simulink model "EIRSAT_ADCS"  (R2017a)
settings: Solver=ode45  StartTime=0.0  StopTime=T_stop  RelTol=1e-6
values from neighbouring files (symbols this model uses):
  aerodrag_A_d = 0.2*0.1*sqrt(2)    [Satellite_Setup.m]
  aerodrag_c_p = 0.02*[1;1;1]    [Satellite_Setup.m]
  I = diag([Ixx;Iyy;Izz])    [Satellite_Setup.m]
  igrf_L = 10    [Satellite_Setup.m]
  igrf_tol = 1e-9    (= 1e-09)    [Satellite_Setup.m]
  mass = 2.6    [Satellite_Setup.m]
  omega_orbit = [0;-7.67/(401.1+6371);0]    [Satellite_Setup.m]
undefined symbols (not defined in the file or in its folder): control_tolerance, distrej, igrf_G, igrf_H, k, kd, kp, nAx, nAy, nAz, q_ref, x_0, x_orbit_init
libraries: cstblocks x12, sharedtransform x4
settings Model: Creator=JoeT  LastModifiedBy=vicctorio
settings DataIOCC: LimitDataPoints=on  SaveFormat=Array
settings OptimizationCC: BlockReduction=off  BooleanDataType=off  LifeSpan=inf
settings DebuggingCC: SaveWithParameterizedLinksMsg=none  UnderspecifiedInitializationDetection=Classic  MergeDetectMultiDrivingBlocksExec=none  SignalResolutionControl=TryResolveAllWithWarning  SFUnexpectedBacktrackingDiag=warning  SFNoUnconditionalDefaultTransitionDiag=warning  SFExecutionAtInitializationDiag=none
settings HardwareCC: ProdBitPerPointer=32  ProdBitPerSizeT=32  ProdBitPerPtrDiffT=32  ProdLargestAtomicFloat=None  ProdIntDivRoundTo=Undefined  ProdEndianess=Unspecified  ProdWordSize=32  ProdHWDeviceType=32-bit Generic  TargetUnknown=on
settings ModelReferenceCC: PropagateSignalLabelsOutOfModel=off
settings GRTTargetCC: TargetLangStandard=C89/C90 (ANSI)  GeneratePreprocessorConditionals=Disable all
settings ConfigComp: CovMetricSettings=dw  CovHtmlReporting=on  CovSaveCumulativeToWorkspaceVar=on  CovSaveSingleToWorkspaceVar=on  CovExternalEMLEnable=off  CovSFcnEnable=off

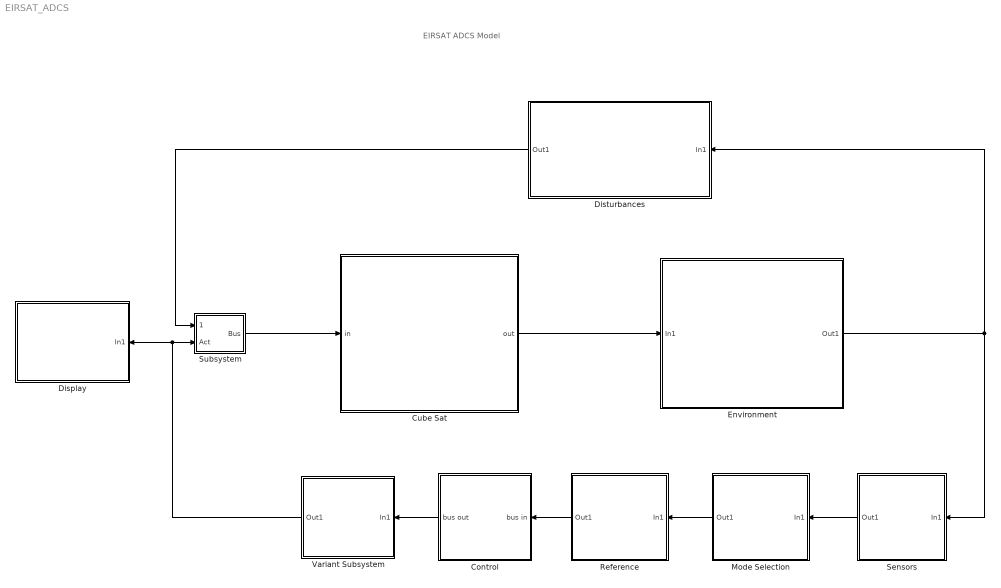
== system EIRSAT_ADCS ==
  note: EIRSAT ADCS Model
  Control : Subsystem  Variant=on
  Cube Sat : Subsystem
  Display : Subsystem
  Disturbances : Subsystem
  Environment : Subsystem
  Mode Selection : Subsystem
  Reference : Subsystem
  Sensors : Subsystem
  Subsystem : Subsystem
  Variant Subsystem : Subsystem  Variant=on
  wires:
  Mode Selection/1(Out1) -> Reference/1(In1)
  Sensors/1(Out1) -> Mode Selection/1(In1)
  Reference/1(Out1) -> Control/1(bus in)
  Control/1(bus out) -> Variant Subsystem/1(In1)
  Disturbances/1(Out1) -> Subsystem/1(Disturb)
  Cube Sat/1(out) -> Environment/1(In1)
  Environment/1(Out1) -> Sensors/1(In1), Disturbances/1(In1)
  Variant Subsystem/1(Out1) -> Subsystem/2(Act), Display/1(In1)
  Subsystem/1(Bus) -> Cube Sat/1(in)

== system EIRSAT_ADCS/Control ==
  note: 1) Only subsystems can be added as variant choices at this level
      | 2) Blocks cannot be connected at this level as connectivity is
      | automatically determined at simulation, based on the active variant
  bus in : Inport
  PD : Subsystem  VariantControl=CtrlType==2
  WBC : Subsystem  VariantControl=CtrlType==1
  no control : Subsystem  VariantControl=CtrlType==0
  bus out : Outport

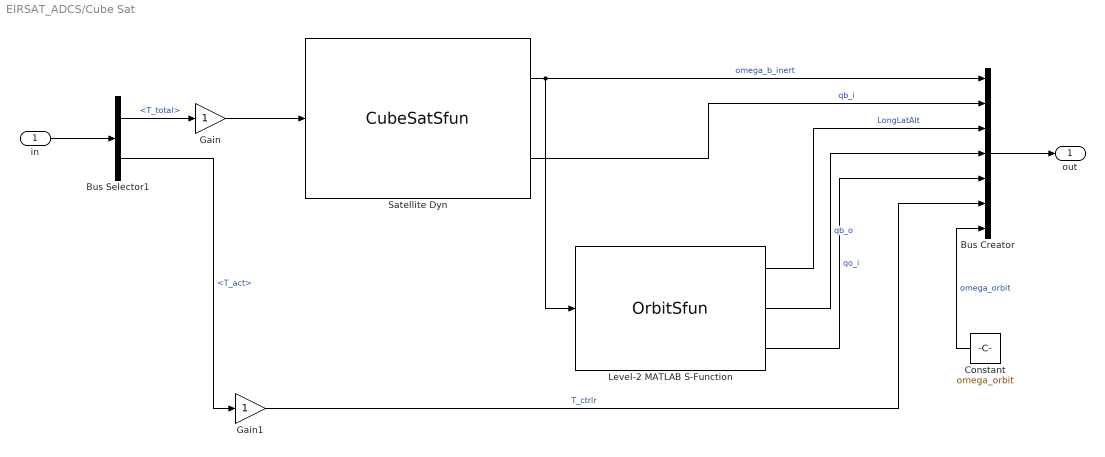
== system EIRSAT_ADCS/Cube Sat ==
  in : Inport
  Bus Creator : BusCreator  Inputs=7
  Bus Selector1 : BusSelector  OutputSignals=T_total,T_act
  Constant : Constant  Value=omega_orbit
  Gain : Gain
  Gain1 : Gain
  Level-2 MATLAB S-Function : M-S-Function  FunctionName=OrbitSfun  Parameters=x_orbit_init,omega_orbit  mask{Parameter1=x_orbit_init, Parameter2=omega_orbit}
      mask prompts: Parameter1 "Initial orbit param"; Parameter2 "orbit angular velocity"
      mask DialogControl Control8 Prompt: Orbit properties
      mask Display:
      | disp('Orbital Parameters')
      | port_label('input',1,'ang vel')
      | port_label('output',1,'LLA')
      | port_label('output',2,'qb_o')
      | port_label('output',3,'qo_i')
  Satellite Dyn : M-S-Function  FunctionName=CubeSatSfun  Parameters=x_0,I  mask{Parameter2=x_0, Parameter3=I}
      mask prompts: Parameter2 "x_0"; Parameter3 "I"
      mask DialogControl DescTextVar Prompt: Model of a rigid CubeSat. Model takes Torque about each axis as an input. The first output is the angular velocity of the sat wrt an inertial frame. The second output is the quaternion which represents the rotation between inertial and body fixed frames
      mask Display:
      | disp('Cube Sat Model')
      | port_label('input',1,'Torq')
      | port_label('output',1,'Ang Vel')
      | port_label('output',2,'Quat')
  out : Outport
  wires:
  Bus Creator/1 -> out/1
  in/1 -> Bus Selector1/1
  Bus Selector1/1 -> Gain/1  "<T_total>"
  Satellite Dyn/1 -> Level-2 MATLAB S-Function/1, Bus Creator/1  "omega_b_inert"
  Gain/1 -> Satellite Dyn/1
  Satellite Dyn/2 -> Bus Creator/2  "qb_i"
  Level-2 MATLAB S-Function/1 -> Bus Creator/3  "LongLatAlt"
  Level-2 MATLAB S-Function/2 -> Bus Creator/4  "qb_o"
  Level-2 MATLAB S-Function/3 -> Bus Creator/5  "qo_i"
  Constant/1 -> Bus Creator/7  "omega_orbit"
  Bus Selector1/2 -> Gain1/1  "<T_act>"
  Gain1/1 -> Bus Creator/6  "T_ctrlr"

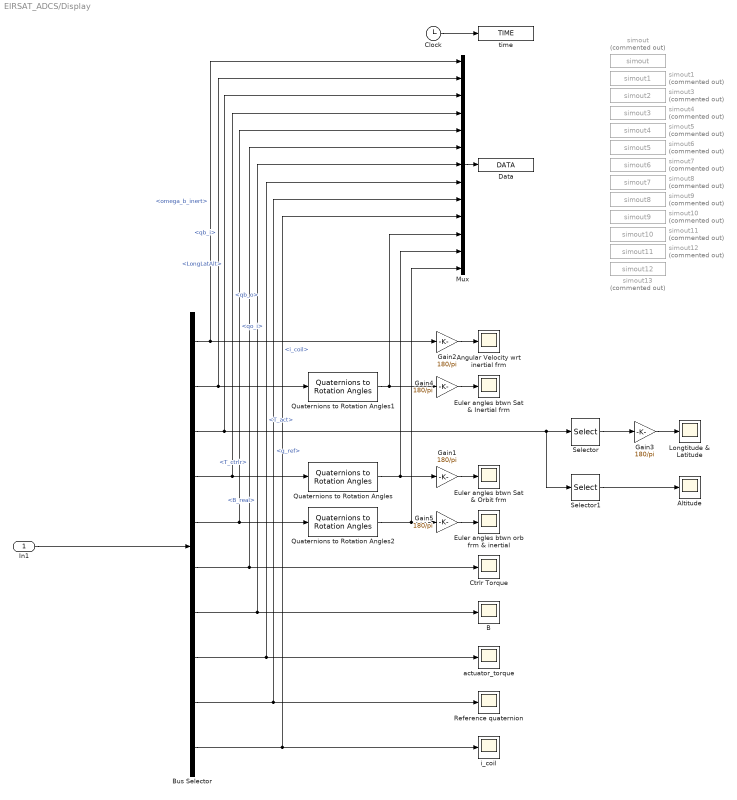
== system EIRSAT_ADCS/Display ==
  In1 : Inport
  Altitude : Scope
  Angular Velocity wrt inertial frm : Scope
  B : Scope
  Bus Selector : BusSelector  OutputSignals=Ctrlr_out.ref_out.signal1.Sensor_out.Enviro_out.Dyn_out.omega_b_inert,Ctrlr_out.ref_out.signal1.Sensor_out.Enviro_out.Dyn_out.qb_i,Ctrlr_out.ref_out.signal1.Sensor_out.Enviro_out.Dyn_out.LongLatAlt,Ctrlr_out.ref_out.signal1.Sensor_out.Enviro_out.Dyn_out.qb_o,Ctrlr_out.ref_out.signal1.Sensor_out.Enviro_out.Dyn_out.qo_i,Ctrlr_out.ref_out.signal1.Sensor_out.Enviro_out.Dyn_out.T_ctrlr,Ctrlr_out.ref_out.signal1.Sensor_out.Sensor_values.B_real,T_act,Ctrlr_out.ref_out.q_ref,i_coil
  Clock : Clock
  Ctrlr Torque : Scope
  "Data " : ToWorkspace  VariableName=DATA  SampleTime=-1
  Euler angles btwn Sat & Inertial frm : Scope
  Euler angles btwn Sat & Orbit frm : Scope
  Euler angles btwn orb frm & inertial : Scope
  Gain{1..5} (5 alike) : Gain  Gain=180/pi
  Longtitude & Latitude : Scope
  Mux : Mux  Inputs=13
  Quaternions to Rotation Angles : sharedtransform/Quaternions to Rotation Angles  rotationOrder=XYZ
  Quaternions to Rotation Angles1 : sharedtransform/Quaternions to Rotation Angles  rotationOrder=XYZ
  Quaternions to Rotation Angles2 : sharedtransform/Quaternions to Rotation Angles  rotationOrder=XYZ
  Reference quaternion : Scope
  Selector : Selector  InputPortWidth=3  IndexOptions=Index vector (dialog)  Indices=[1 2]  OutputSizes=1
  Selector1 : Selector  InputPortWidth=3  IndexOptions=Index vector (dialog)  Indices=[3]  OutputSizes=1
  actuator_torque : Scope
  i_coil : Scope
  "simout " : ToWorkspace  Commented=on  VariableName=simout  SaveFormat=Timeseries  SampleTime=-1
  simout1 : ToWorkspace  Commented=on  VariableName=simout1  SaveFormat=Timeseries  SampleTime=-1
  simout10 : ToWorkspace  Commented=on  VariableName=simout9  SaveFormat=Timeseries  SampleTime=-1
  simout11 : ToWorkspace  Commented=on  VariableName=simout10  SaveFormat=Timeseries  SampleTime=-1
  simout12 : ToWorkspace  Commented=on  VariableName=simout11  SaveFormat=Timeseries  SampleTime=-1
  simout13 : ToWorkspace  Commented=on  VariableName=simout12  SaveFormat=Timeseries  SampleTime=-1
  simout3 : ToWorkspace  Commented=on  VariableName=simout2  SaveFormat=Timeseries  SampleTime=-1
  simout4 : ToWorkspace  Commented=on  VariableName=simout3  SaveFormat=Timeseries  SampleTime=-1
  simout5 : ToWorkspace  Commented=on  VariableName=simout4  SaveFormat=Timeseries  SampleTime=-1
  simout6 : ToWorkspace  Commented=on  VariableName=simout5  SaveFormat=Timeseries  SampleTime=-1
  simout7 : ToWorkspace  Commented=on  VariableName=simout6  SaveFormat=Timeseries  SampleTime=-1
  simout8 : ToWorkspace  Commented=on  VariableName=simout7  SaveFormat=Timeseries  SampleTime=-1
  simout9 : ToWorkspace  Commented=on  VariableName=simout8  SaveFormat=Timeseries  SampleTime=-1
  time : ToWorkspace  VariableName=TIME  SampleTime=-1
  wires:
  In1/1 -> Bus Selector/1
  Bus Selector/6 -> Mux/6, Ctrlr Torque/1  "<T_ctrlr>"
  Bus Selector/4 -> Mux/4, Quaternions to Rotation Angles/1  "<qb_o>"
  Bus Selector/1 -> Mux/1, Gain2/1  "<omega_b_inert>"
  Quaternions to Rotation Angles/1 -> Mux/12, Gain1/1
  Gain2/1 -> Angular Velocity wrt inertial frm/1
  Gain1/1 -> Euler angles btwn Sat & Orbit frm/1
  Selector/1 -> Gain3/1
  Gain3/1 -> Longtitude & Latitude/1
  Bus Selector/2 -> Mux/2, Quaternions to Rotation Angles1/1  "<qb_i>"
  Selector1/1 -> Altitude/1
  Quaternions to Rotation Angles2/1 -> Mux/13, Gain5/1
  Gain5/1 -> Euler angles btwn orb frm & inertial/1
  Bus Selector/3 -> Mux/3, Selector1/1, Selector/1  "<LongLatAlt>"
  Bus Selector/7 -> Mux/7, B/1  "<B_real>"
  Bus Selector/8 -> Mux/8, actuator_torque/1  "<T_act>"
  Bus Selector/9 -> Mux/9, Reference quaternion/1  "<q_ref>"
  Bus Selector/10 -> Mux/10, i_coil/1  "<i_coil>"
  Gain4/1 -> Euler angles btwn Sat & Inertial frm/1
  Bus Selector/5 -> Mux/5, Quaternions to Rotation Angles2/1  "<qo_i>"
  Quaternions to Rotation Angles1/1 -> Mux/11, Gain4/1
  Mux/1 -> "Data "/1
  Clock/1 -> time/1

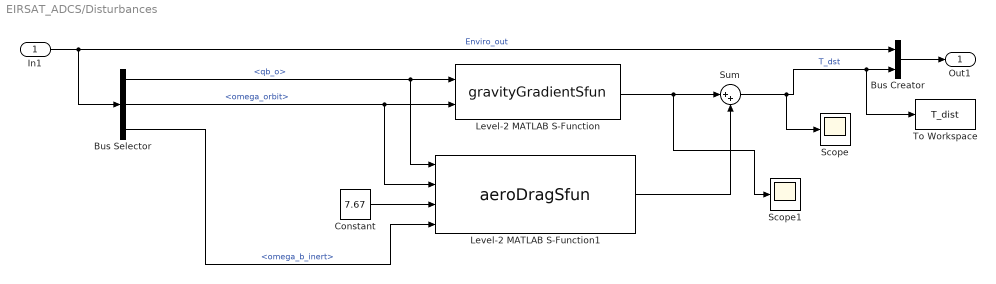
== system EIRSAT_ADCS/Disturbances ==
  In1 : Inport
  Bus Creator : BusCreator  Inputs=2
  Bus Selector : BusSelector  OutputSignals=Dyn_out.qb_o,Dyn_out.omega_orbit,Dyn_out.omega_b_inert
  Constant : Constant  Value=7.67
  Level-2 MATLAB S-Function : M-S-Function  FunctionName=gravityGradientSfun
      mask Display:
      | disp('Gravity\n gradient')
      | port_label('input',1,'qb_o')
      | port_label('input',2,'omega orbit')
      | port_label('output',1,'T_b')
  Level-2 MATLAB S-Function1 : M-S-Function  FunctionName=aeroDragSfun  Parameters=I,mass,aerodrag_c_p,aerodrag_A_d  mask{Parameter1=I, Parameter2=mass, Parameter3=aerodrag_c_p, Parameter4=aerodrag_A_d}
      mask prompts: Parameter1 "Inertia"; Parameter2 "Mass"; Parameter3 "COP vector"; Parameter4 "Area"
      mask Display:
      | disp('Aerodynamic\n drag')
      | port_label('input',1,'qb_o')
      | port_label('input',2,'omega orbit')
      | port_label('input',3,'Local atmosph. vel')
      | port_label('output',1,'T_b')
  Scope : Scope
  Scope1 : Scope
  Sum : Sum  Inputs=|++
  To Workspace : ToWorkspace  VariableName=T_dist  SampleTime=-1
  Out1 : Outport
  wires:
  Level-2 MATLAB S-Function/1 -> Scope1/1, Sum/1
  Level-2 MATLAB S-Function1/1 -> Sum/2
  In1/1 -> Bus Creator/1, Bus Selector/1  "Enviro_out"
  Bus Selector/1 -> Level-2 MATLAB S-Function1/1, Level-2 MATLAB S-Function/1  "<qb_o>"
  Bus Selector/2 -> Level-2 MATLAB S-Function/2, Level-2 MATLAB S-Function1/2  "<omega_orbit>"
  Constant/1 -> Level-2 MATLAB S-Function1/3
  Sum/1 -> To Workspace/1, Bus Creator/2, Scope/1  "T_dst"
  Bus Selector/3 -> Level-2 MATLAB S-Function1/4  "<omega_b_inert>"
  Bus Creator/1 -> Out1/1

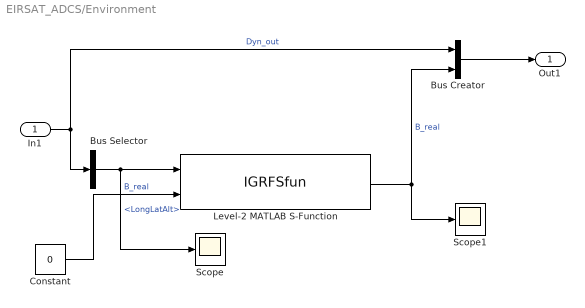
== system EIRSAT_ADCS/Environment ==
  In1 : Inport
  Bus Creator : BusCreator  Inputs=2
  Bus Selector : BusSelector  OutputSignals=LongLatAlt
  Constant : Constant  Value=0
  Level-2 MATLAB S-Function : M-S-Function  FunctionName=IGRFSfun  Parameters=igrf_L,igrf_tol,igrf_G,igrf_H  mask{Parameter1=igrf_L, Parameter2=igrf_tol, Parameter3=igrf_G, Parameter4=igrf_H}
      mask prompts: Parameter1 "L"; Parameter2 "tolerance"; Parameter3 "G_coefs"; Parameter4 "H_coefs"
      mask Display:
      | disp('IGRF\n  Geomagnetic reference')
      | port_label('input',1,'LLA')
      | port_label('output',1,'real B')
  Scope : Scope
  Scope1 : Scope
  Out1 : Outport
  wires:
  In1/1 -> Bus Creator/1, Bus Selector/1  "Dyn_out"
  Bus Selector/1 -> Scope/1, Level-2 MATLAB S-Function/1  "<LongLatAlt>"
  Level-2 MATLAB S-Function/1 -> Bus Creator/2, Scope1/1  "B_real"
  Bus Creator/1 -> Out1/1
  Constant/1 -> Level-2 MATLAB S-Function/2  "B_real"

== system EIRSAT_ADCS/Mode Selection ==
  In1 : Inport
  Bus Creator : BusCreator  Inputs=2
  Constant : Constant
  Out1 : Outport
  wires:
  In1/1 -> Bus Creator/1  "Sensor_out"
  Bus Creator/1 -> Out1/1
  Constant/1 -> Bus Creator/2  "mode"

== system EIRSAT_ADCS/Reference ==
  In1 : Inport
  Bus Creator : BusCreator  Inputs=2
  Constant : Constant  Value=q_ref
  Out1 : Outport
  wires:
  In1/1 -> Bus Creator/1
  Bus Creator/1 -> Out1/1
  Constant/1 -> Bus Creator/2  "q_ref"

== system EIRSAT_ADCS/Sensors ==
  In1 : Inport
  Bus Creator : BusCreator  Inputs=2
  Bus Selector : BusSelector  OutputSignals=B_real,Dyn_out.LongLatAlt,Dyn_out.qb_i,Dyn_out.omega_b_inert  OutputAsBus=on
  Out1 : Outport
  wires:
  In1/1 -> Bus Selector/1, Bus Creator/1  "Enviro_out"
  Bus Creator/1 -> Out1/1
  Bus Selector/1 -> Bus Creator/2  "Sensor_values"

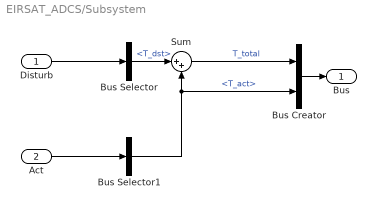
== system EIRSAT_ADCS/Subsystem ==
  Disturb : Inport
  Act : Inport  Port=2
  Bus Creator : BusCreator  Inputs=2
  Bus Selector : BusSelector  OutputSignals=T_dst
  Bus Selector1 : BusSelector  OutputSignals=T_act
  Sum : Sum  Inputs=|++
  Bus : Outport
  wires:
  Disturb/1 -> Bus Selector/1
  Act/1 -> Bus Selector1/1
  Bus Selector/1 -> Sum/1  "<T_dst>"
  Sum/1 -> Bus Creator/1  "T_total"
  Bus Selector1/1 -> Sum/2, Bus Creator/2  "<T_act>"
  Bus Creator/1 -> Bus/1

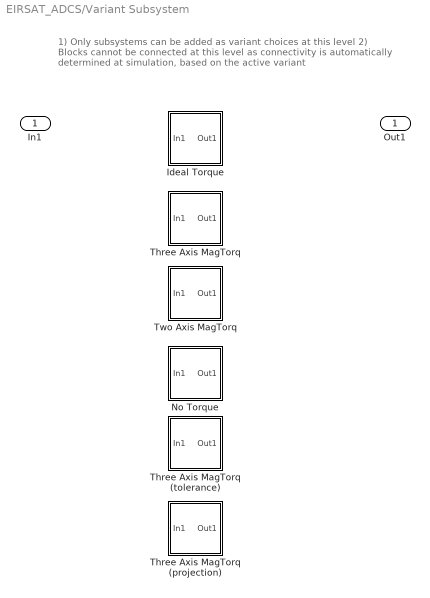
== system EIRSAT_ADCS/Variant Subsystem ==
  note: 1) Only subsystems can be added as variant choices at this level
      | 2) Blocks cannot be connected at this level as connectivity is
      | automatically determined at simulation, based on the active variant
  In1 : Inport
  Ideal Torque : Subsystem  VariantControl=ActType==1
  No Torque : Subsystem  VariantControl=ActType==4
  Three Axis MagTorq : Subsystem  VariantControl=ActType==2
  Three Axis MagTorq (projection) : Subsystem  VariantControl=ActType==6
  Three Axis MagTorq (tolerance) : Subsystem  VariantControl=ActType==5
  Two Axis MagTorq : Subsystem  VariantControl=ActType==3
  Out1 : Outport

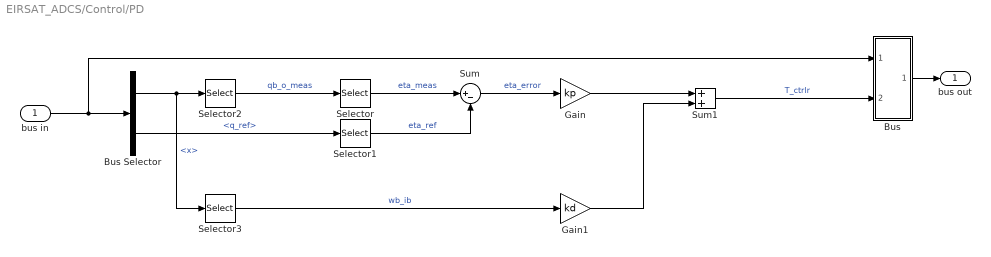
== system EIRSAT_ADCS/Control/PD ==
  bus in : Inport
  Bus : Subsystem
  Bus Selector : BusSelector  OutputSignals=Sensor_out.x,q_ref
  Gain : Gain  Gain=kp
  Gain1 : Gain  Gain=kd
  Selector : Selector  InputPortWidth=4  IndexOptions=Index vector (dialog)  Indices=[2 3 4]  OutputSizes=1
  Selector1 : Selector  InputPortWidth=4  IndexOptions=Index vector (dialog)  Indices=[2 3 4]  OutputSizes=1
  Selector2 : Selector  InputPortWidth=18  IndexOptions=Index vector (dialog)  Indices=[4;5;6;7]  OutputSizes=1
  Selector3 : Selector  InputPortWidth=18  IndexOptions=Index vector (dialog)  Indices=[1,2,3]  OutputSizes=1
  Sum : Sum  Inputs=|+-
  Sum1 : Sum
  bus out : Outport
  wires:
  bus in/1 -> Bus/1(In1), Bus Selector/1
  Bus Selector/2 -> Selector1/1  "<q_ref>"
  Selector2/1 -> Selector/1  "qb_o_meas"
  Bus Selector/1 -> Selector3/1, Selector2/1  "<x>"
  Selector/1 -> Sum/1  "eta_meas"
  Selector1/1 -> Sum/2  "eta_ref"
  Sum/1 -> Gain/1  "eta_error"
  Gain/1 -> Sum1/1
  Selector3/1 -> Gain1/1  "wb_ib"
  Gain1/1 -> Sum1/2
  Bus/1(Out1) -> bus out/1
  Sum1/1 -> Bus/2(In2)  "T_ctrlr"

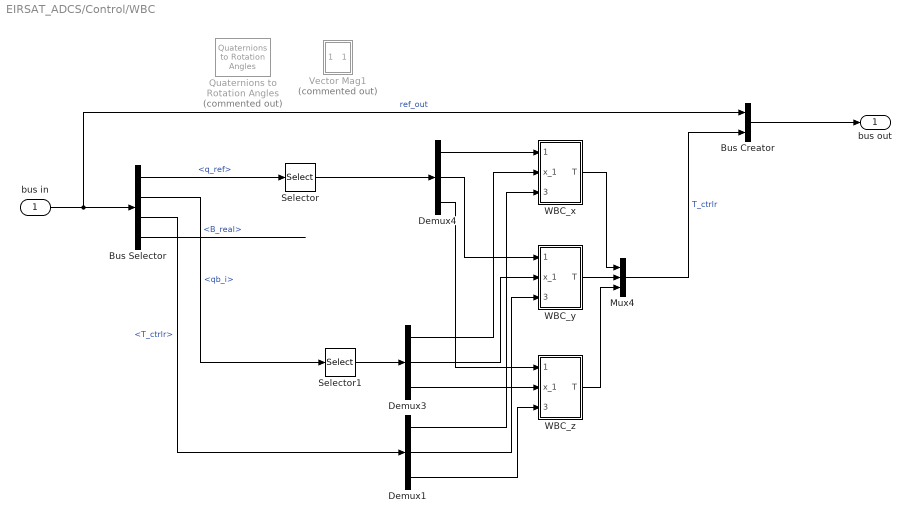
== system EIRSAT_ADCS/Control/WBC ==
  bus in : Inport
  Bus Creator : BusCreator  Inputs=2
  Bus Selector : BusSelector  OutputSignals=q_ref,signal1.Sensor_out.Enviro_out.Dyn_out.qb_i,signal1.Sensor_out.Enviro_out.Dyn_out.T_ctrlr,signal1.Sensor_out.Sensor_values.B_real
  Demux1 : Demux  Outputs=3
  Demux3 : Demux  Outputs=3
  Demux4 : Demux  Outputs=3
  Mux4 : Mux  Inputs=3
  Quaternions to Rotation Angles : sharedtransform/Quaternions to Rotation Angles  Commented=on  rotationOrder=XZY
      settings: SourceProductBaseCode=AE
  Selector : Selector  InputPortWidth=4  IndexOptions=Index vector (dialog)  Indices=[2 3 4]  OutputSizes=1
  Selector1 : Selector  InputPortWidth=4  IndexOptions=Index vector (dialog)  Indices=[2 3 4]  OutputSizes=1
  Vector Mag1 : Subsystem  Commented=on
  WBC_x : Subsystem
  WBC_y : Subsystem
  WBC_z : Subsystem
  bus out : Outport
  wires:
  Demux3/3 -> WBC_z/2(x_1)
  WBC_y/1(T) -> Mux4/2
  Mux4/1 -> Bus Creator/2  "T_ctrlr"
  WBC_z/1(T) -> Mux4/3
  WBC_x/1(T) -> Mux4/1
  Demux3/2 -> WBC_y/2(x_1)
  Demux3/1 -> WBC_x/2(x_1)
  Bus Selector/3 -> Demux1/1  "<T_ctrlr>"
  Demux1/1 -> WBC_x/3(T_meas)
  Demux1/2 -> WBC_y/3(T_meas)
  Demux1/3 -> WBC_z/3(T_meas)
  Demux4/1 -> WBC_x/1(x_0_ref)
  Demux4/3 -> WBC_z/1(x_0_ref)
  Demux4/2 -> WBC_y/1(x_0_ref)
  Selector1/1 -> Demux3/1
  bus in/1 -> Bus Creator/1, Bus Selector/1  "ref_out"
  Bus Selector/1 -> Selector/1  "<q_ref>"
  Bus Selector/2 -> Selector1/1  "<qb_i>"
  Bus Creator/1 -> bus out/1
  Bus Selector/4 -> ?  "<B_real>"
  Selector/1 -> Demux4/1

== system EIRSAT_ADCS/Control/no control ==
  bus in : Inport
  Bus : Subsystem  Commented=on
  Bus Creator : BusCreator  Inputs=2
  Constant : Constant  Value=[0;0;0]
  bus out : Outport
  wires:
  bus in/1 -> Bus Creator/1  "ref_out"
  Constant/1 -> Bus Creator/2  "T_ctrlr"
  Bus Creator/1 -> bus out/1

== system EIRSAT_ADCS/Variant Subsystem/Ideal Torque ==
  In1 : Inport
  Bus Creator : BusCreator  Inputs=2
  Bus Selector : BusSelector  OutputSignals=T_ctrlr
  Gain : Gain
  Out1 : Outport
  wires:
  In1/1 -> Bus Selector/1, Bus Creator/1  "Ctrlr_out"
  Bus Creator/1 -> Out1/1
  Bus Selector/1 -> Gain/1  "<T_ctrlr>"
  Gain/1 -> Bus Creator/2  "T_act"

== system EIRSAT_ADCS/Variant Subsystem/No Torque ==
  In1 : Inport
  Bus Creator : BusCreator  Inputs=2
  Bus Selector : BusSelector  OutputSignals=T_ctrlr
  Gain : Gain  Gain=0
  Out1 : Outport
  wires:
  Gain/1 -> Bus Creator/2  "T_act"
  Bus Selector/1 -> Gain/1  "<T_ctrlr>"
  Bus Creator/1 -> Out1/1
  In1/1 -> Bus Creator/1, Bus Selector/1  "Ctrlr_out"

== system EIRSAT_ADCS/Variant Subsystem/Three Axis MagTorq ==
  In1 : Inport
  Bus Creator : BusCreator  Inputs=4
  Bus Selector : BusSelector  OutputSignals=T_ctrlr,ref_out.signal1.Sensor_out.Enviro_out.B_real,ref_out.signal1.Sensor_out.Sensor_values.B_real
  Level-2 MATLAB S-Function : M-S-Function  FunctionName=Magtorq2Sfun  Parameters=nAx, nAy, nAz
  Out1 : Outport
  wires:
  In1/1 -> Bus Selector/1, Bus Creator/1  "Ctrlr_out"
  Bus Creator/1 -> Out1/1
  Bus Selector/3 -> Level-2 MATLAB S-Function/3  "<B_real>"
  Level-2 MATLAB S-Function/1 -> Bus Creator/2  "T_act"
  Bus Selector/1 -> Level-2 MATLAB S-Function/1  "<T_ctrlr>"
  Bus Selector/2 -> Level-2 MATLAB S-Function/2  "<B_real>"
  Level-2 MATLAB S-Function/2 -> Bus Creator/3  "m_coil"
  Level-2 MATLAB S-Function/3 -> Bus Creator/4  "i_coil"

== system EIRSAT_ADCS/Variant Subsystem/Three Axis MagTorq (projection) ==
  In1 : Inport
  Bus Creator : BusCreator  Inputs=4
  Bus Selector : BusSelector  OutputSignals=T_ctrlr,ref_out.signal1.Sensor_out.Enviro_out.B_real,ref_out.signal1.Sensor_out.Sensor_values.B_real
  Level-2 MATLAB S-Function : M-S-Function  FunctionName=Magtorq4Sfun  Parameters=nAx,nAy,nAz
  Out1 : Outport
  wires:
  In1/1 -> Bus Selector/1, Bus Creator/1  "Ctrlr_out"
  Bus Creator/1 -> Out1/1
  Bus Selector/3 -> Level-2 MATLAB S-Function/3  "<B_real>"
  Level-2 MATLAB S-Function/1 -> Bus Creator/2  "T_act"
  Bus Selector/1 -> Level-2 MATLAB S-Function/1  "<T_ctrlr>"
  Bus Selector/2 -> Level-2 MATLAB S-Function/2  "<B_real>"
  Level-2 MATLAB S-Function/2 -> Bus Creator/3  "m_coil"
  Level-2 MATLAB S-Function/3 -> Bus Creator/4  "i_coil"

== system EIRSAT_ADCS/Variant Subsystem/Three Axis MagTorq (tolerance) ==
  In1 : Inport
  Bus Creator : BusCreator  Inputs=4
  Bus Selector : BusSelector  OutputSignals=T_ctrlr,ref_out.signal1.Sensor_out.Enviro_out.B_real,ref_out.signal1.Sensor_out.Sensor_values.B_real
  Level-2 MATLAB S-Function : M-S-Function  FunctionName=Magtorq3Sfun  Parameters=control_tolerance,nAx,nAy,nAz
  Out1 : Outport
  wires:
  In1/1 -> Bus Selector/1, Bus Creator/1  "Ctrlr_out"
  Bus Creator/1 -> Out1/1
  Bus Selector/3 -> Level-2 MATLAB S-Function/3  "<B_real>"
  Level-2 MATLAB S-Function/1 -> Bus Creator/2  "T_act"
  Bus Selector/1 -> Level-2 MATLAB S-Function/1  "<T_ctrlr>"
  Bus Selector/2 -> Level-2 MATLAB S-Function/2  "<B_real>"
  Level-2 MATLAB S-Function/2 -> Bus Creator/3  "m_coil"
  Level-2 MATLAB S-Function/3 -> Bus Creator/4  "i_coil"

== system EIRSAT_ADCS/Variant Subsystem/Two Axis MagTorq ==
  In1 : Inport
  Bus Creator : BusCreator  Inputs=4
  Bus Selector : BusSelector  OutputSignals=T_ctrlr,ref_out.Mode_select_out.Sensor_out.Enviro_out.B_real,ref_out.Mode_select_out.Sensor_out.Sensor_values.B_real
  Level-2 MATLAB S-Function : M-S-Function  FunctionName=MagtorqSfun
  Selector : Selector  InputPortWidth=3  IndexOptions=Index vector (dialog)  Indices=[1 2]  OutputSizes=1
  Out1 : Outport
  wires:
  In1/1 -> Bus Selector/1, Bus Creator/1
  Bus Creator/1 -> Out1/1
  Bus Selector/3 -> Level-2 MATLAB S-Function/3  "<B_real>"
  Bus Selector/1 -> Level-2 MATLAB S-Function/1  "<T_ctrlr>"
  Bus Selector/2 -> Level-2 MATLAB S-Function/2  "<B_real>"
  Level-2 MATLAB S-Function/1 -> Selector/1
  Selector/1 -> Bus Creator/2  "m_coils"
  Level-2 MATLAB S-Function/2 -> Bus Creator/3
  ? -> Bus Creator/4  "i_coil"

== system EIRSAT_ADCS/Control/PD/Bus ==
  In1 : Inport
  In2 : Inport  Port=2
  Bus Creator : BusCreator  Inputs=9
  Bus Selector1 : BusSelector  OutputSignals=Mode_select_out.signal1.Dyn_out.omega_b_inert,Mode_select_out.signal1.Dyn_out.qb_i,Mode_select_out.signal1.Dyn_out.LongLatAlt,Mode_select_out.signal1.Dyn_out.qb_o,Mode_select_out.signal1.Dyn_out.qo_i,Mode_select_out.signal1.Dyn_out.omega_orbit,Mode_select_out.signal1.Dyn_out.T_ctrlr,Mode_select_out.signal1.B_real
  Out1 : Outport
  wires:
  In1/1 -> Bus Selector1/1
  Bus Creator/1 -> Out1/1
  Bus Selector1/1 -> Bus Creator/1  "<omega_b_inert>"
  Bus Selector1/2 -> Bus Creator/2  "<qb_i>"
  Bus Selector1/3 -> Bus Creator/3  "<LongLatAlt>"
  Bus Selector1/4 -> Bus Creator/4  "<qb_o>"
  Bus Selector1/5 -> Bus Creator/5  "<qo_i>"
  Bus Selector1/6 -> Bus Creator/6  "<omega_orbit>"
  Bus Selector1/7 -> Bus Creator/7  "<T_ctrlr>"
  Bus Selector1/8 -> Bus Creator/8  "<B_real>"
  In2/1 -> Bus Creator/9  "T_ctrlr"

== system EIRSAT_ADCS/Control/WBC/Vector Mag1 ==
  v : Inport
  Math Function2 : Math  Operator=square  SaturateOnIntegerOverflow=on
  Sqrt2 : Sqrt  SaturateOnIntegerOverflow=on
  Sum2 : Sum  Inputs=+
  m : Outport
  wires:
  Sqrt2/1 -> m/1
  v/1 -> Math Function2/1
  Math Function2/1 -> Sum2/1
  Sum2/1 -> Sqrt2/1

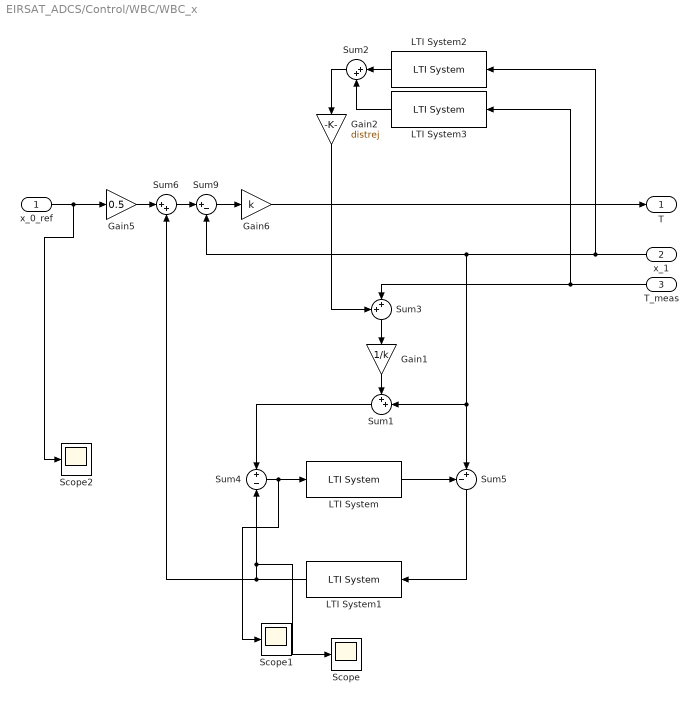
== system EIRSAT_ADCS/Control/WBC/WBC_x ==
  x_0_ref : Inport
  x_1 : Inport  Port=2
  T_meas : Inport  Port=3
  Gain1 : Gain  Gain=1/k
  Gain2 : Gain  Gain=distrej
  Gain5 : Gain  Gain=0.5
  Gain6 : Gain  Gain=k
  LTI System : cstblocks/LTI System  sys=G  IC=[]
  LTI System1 : cstblocks/LTI System  sys=G  IC=[]
  LTI System2 : cstblocks/LTI System  sys=tf(1,[1 1])  IC=[]
  LTI System3 : cstblocks/LTI System  sys=tf(1,[1 1])  IC=[]
  Scope : Scope
  Scope1 : Scope
  Scope2 : Scope
  Sum1 : Sum  Inputs=++|
  Sum2 : Sum  Inputs=|++
  Sum3 : Sum  Inputs=++|
  Sum4 : Sum  Inputs=+|-
  Sum5 : Sum  Inputs=-+|
  Sum6 : Sum  Inputs=|++
  Sum9 : Sum  Inputs=|+-
  T : Outport
  wires:
  Sum1/1 -> Sum4/1
  Gain1/1 -> Sum1/1
  x_1/1 -> Sum1/2, Sum5/2, Sum9/2, LTI System2/1
  Sum5/1 -> LTI System1/1
  LTI System/1 -> Sum5/1
  Sum4/1 -> Scope1/1, LTI System/1
  LTI System1/1 -> Scope/1, Sum4/2, Sum6/2
  Gain5/1 -> Sum6/1
  Gain6/1 -> T/1
  Sum9/1 -> Gain6/1
  Sum6/1 -> Sum9/1
  LTI System2/1 -> Sum2/1
  LTI System3/1 -> Sum2/2
  Sum2/1 -> Gain2/1
  Sum3/1 -> Gain1/1
  Gain2/1 -> Sum3/1
  T_meas/1 -> Sum3/2, LTI System3/1
  x_0_ref/1 -> Scope2/1, Gain5/1

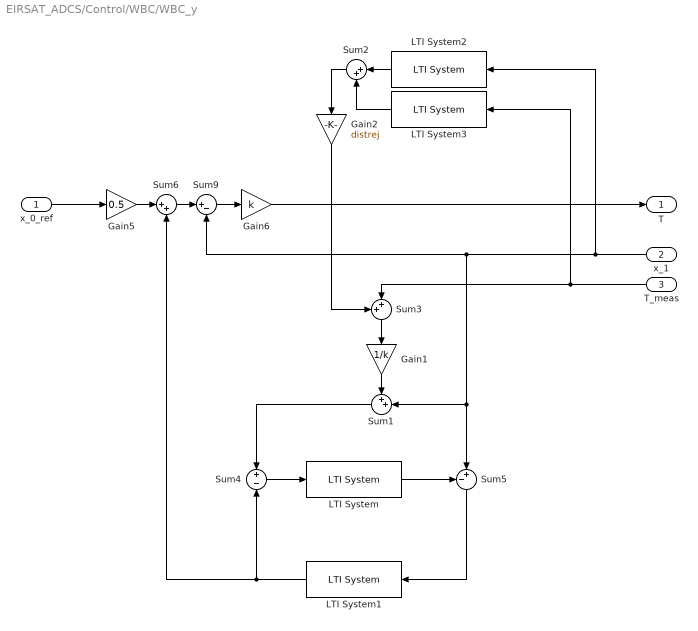
== system EIRSAT_ADCS/Control/WBC/WBC_y ==
  x_0_ref : Inport
  x_1 : Inport  Port=2
  T_meas : Inport  Port=3
  Gain1 : Gain  Gain=1/k
  Gain2 : Gain  Gain=distrej
  Gain5 : Gain  Gain=0.5
  Gain6 : Gain  Gain=k
  LTI System : cstblocks/LTI System  sys=G  IC=[]
  LTI System1 : cstblocks/LTI System  sys=G  IC=[]
  LTI System2 : cstblocks/LTI System  sys=tf(1,[1 1])  IC=[]
  LTI System3 : cstblocks/LTI System  sys=tf(1,[1 1])  IC=[]
  Sum1 : Sum  Inputs=++|
  Sum2 : Sum  Inputs=|++
  Sum3 : Sum  Inputs=++|
  Sum4 : Sum  Inputs=+|-
  Sum5 : Sum  Inputs=-+|
  Sum6 : Sum  Inputs=|++
  Sum9 : Sum  Inputs=|+-
  T : Outport
  wires:
  T_meas/1 -> LTI System3/1, Sum3/2
  x_0_ref/1 -> Gain5/1
  Gain2/1 -> Sum3/1
  Sum3/1 -> Gain1/1
  Sum2/1 -> Gain2/1
  LTI System3/1 -> Sum2/2
  LTI System2/1 -> Sum2/1
  Sum6/1 -> Sum9/1
  Sum9/1 -> Gain6/1
  Gain6/1 -> T/1
  Gain5/1 -> Sum6/1
  LTI System1/1 -> Sum6/2, Sum4/2
  Sum4/1 -> LTI System/1
  LTI System/1 -> Sum5/1
  Sum5/1 -> LTI System1/1
  x_1/1 -> LTI System2/1, Sum9/2, Sum5/2, Sum1/2
  Gain1/1 -> Sum1/1
  Sum1/1 -> Sum4/1

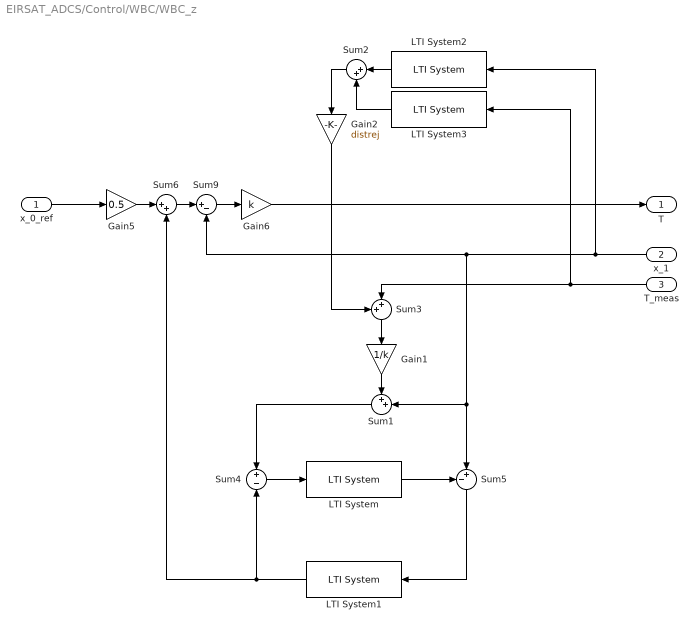
== system EIRSAT_ADCS/Control/WBC/WBC_z ==
  x_0_ref : Inport
  x_1 : Inport  Port=2
  T_meas : Inport  Port=3
  Gain1 : Gain  Gain=1/k
  Gain2 : Gain  Gain=distrej
  Gain5 : Gain  Gain=0.5
  Gain6 : Gain  Gain=k
  LTI System : cstblocks/LTI System  sys=G  IC=[]
  LTI System1 : cstblocks/LTI System  sys=G  IC=[]
  LTI System2 : cstblocks/LTI System  sys=tf(1,[1 1])  IC=[]
  LTI System3 : cstblocks/LTI System  sys=tf(1,[1 1])  IC=[]
  Sum1 : Sum  Inputs=++|
  Sum2 : Sum  Inputs=|++
  Sum3 : Sum  Inputs=++|
  Sum4 : Sum  Inputs=+|-
  Sum5 : Sum  Inputs=-+|
  Sum6 : Sum  Inputs=|++
  Sum9 : Sum  Inputs=|+-
  T : Outport
  wires:
  Sum1/1 -> Sum4/1
  Gain1/1 -> Sum1/1
  x_1/1 -> Sum1/2, Sum5/2, Sum9/2, LTI System2/1
  Sum5/1 -> LTI System1/1
  LTI System/1 -> Sum5/1
  Sum4/1 -> LTI System/1
  LTI System1/1 -> Sum4/2, Sum6/2
  Gain5/1 -> Sum6/1
  Gain6/1 -> T/1
  Sum9/1 -> Gain6/1
  Sum6/1 -> Sum9/1
  LTI System2/1 -> Sum2/1
  LTI System3/1 -> Sum2/2
  Sum2/1 -> Gain2/1
  Sum3/1 -> Gain1/1
  Gain2/1 -> Sum3/1
  x_0_ref/1 -> Gain5/1
  T_meas/1 -> Sum3/2, LTI System3/1

== system EIRSAT_ADCS/Control/no control/Bus ==
  In1 : Inport
  In2 : Inport  Port=2
  Bus Creator : BusCreator  Inputs=10
  Bus Selector1 : BusSelector  OutputSignals=omega_b_inert,qb_i,LongLatAlt,qb_o,qo_i,omega_orbit,T_ctrlr_meas,B_real,q_ref
  Out1 : Outport
  wires:
  In1/1 -> Bus Selector1/1
  Bus Creator/1 -> Out1/1
  Bus Selector1/1 -> Bus Creator/1  "<omega_b_inert>"
  Bus Selector1/2 -> Bus Creator/2  "<qb_i>"
  Bus Selector1/3 -> Bus Creator/3  "<LongLatAlt>"
  Bus Selector1/4 -> Bus Creator/4  "<qb_o>"
  Bus Selector1/5 -> Bus Creator/5  "<qo_i>"
  Bus Selector1/6 -> Bus Creator/6  "<omega_orbit>"
  Bus Selector1/7 -> Bus Creator/7  "<T_ctrlr_meas>"
  Bus Selector1/8 -> Bus Creator/8  "<B_real>"
  In2/1 -> Bus Creator/10  "T_ctrlr"
  Bus Selector1/9 -> Bus Creator/9  "<q_ref>"
